simulink model "hyg"  (R2023b)
settings: Solver=VariableStepAuto  StartTime=0.0  StopTime=10.0  RelTol=1e-3
settings Model: Creator=Admin  LastModifiedBy=Admin

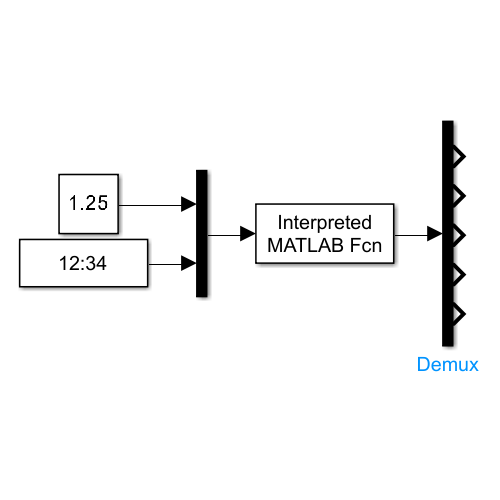
[thumbnail: Simulink's stored preview of the top-level diagram]
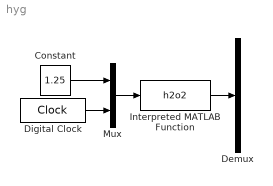
== system hyg ==
  Constant : Constant  Value=1.25
  Demux : Demux  Outputs=5
  Digital Clock : DigitalClock  SampleTime=0.1
  Interpreted MATLAB Function : MATLABFcn  MATLABFcn=h2o2  OutputDimensions=5  Output1D=off
  Mux : Mux  Inputs=2
  wires:
  Constant/1 -> Mux/1
  Digital Clock/1 -> Mux/2
  Mux/1 -> Interpreted MATLAB Function/1
  Interpreted MATLAB Function/1 -> Demux/1
